simulink model "BASK"  (R2023a)
settings: Solver=VariableStepAuto  StartTime=0.0  StopTime=.04  RelTol=1e-3

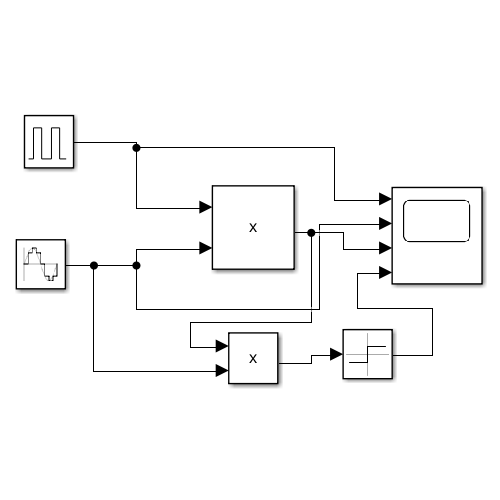
[thumbnail: Simulink's stored preview of the top-level diagram]
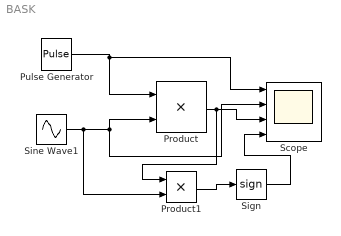
== system BASK ==
  Product : Product
  Product1 : Product
  Pulse Generator : DiscretePulseGenerator  PulseType=Time based  Period=0.01  PulseWidth=50
  Scope : Scope  NumInputPorts=4
  Sign : Signum
  Sine Wave1 : Sin  Frequency=2*pi*1000  SampleTime=0.000001
  wires:
  Sine Wave1/1 -> Product1/2, Product/2, Scope/2
  Pulse Generator/1 -> Product/1, Scope/1
  Product/1 -> Product1/1, Scope/3
  Sign/1 -> Scope/4
  Product1/1 -> Sign/1
